simulink model "OutputToVisualizationContinuous"  (R2016b)
settings: Solver=FixedStepDiscrete  StartTime=0.0  StopTime=10.0  FixedStep=sCoreParams.core.stepPeriod  RelTol=1e-3  EnableMultiTasking=on
undefined symbols (not defined in the file): Low, sCoreParams, sCoreParams_viz_channelInds
libraries: dspswit3 x4, simulink x3, xpcrtudplib x2, slrtlib x2, xpcutilitieslib x1, xpcobsoletelib x1
settings Model: DataTypeOverride=Double  MinMaxOverflowLogging=ForceOff  Creator=rzelmann  LastModifiedBy=rzelmann
settings SolverCC: EnableConcurrentExecution=on  ConcurrentTasks=on  AutoInsertRateTranBlk=on
settings DataIOCC: SaveFormat=StructureWithTime  SaveOutput=off  SignalLogging=off  DSMLogging=off  SaveTime=off
settings OptimizationCC: BlockReduction=off  DefaultParameterBehavior=Inlined  LifeSpan=inf
settings DebuggingCC: AllowSymbolicDim=off  SFUnexpectedBacktrackingDiag=warning  SFNoUnconditionalDefaultTransitionDiag=warning  SFExecutionAtInitializationDiag=none
settings HardwareCC: ProdBitPerPointer=32  ProdBitPerSizeT=32  ProdBitPerPtrDiffT=32  ProdLargestAtomicFloat=None  ProdWordSize=32  ProdLongLongMode=on  ProdHWDeviceType=Generic->32-bit x86 compatible
settings ModelReferenceCC: UpdateModelReferenceTargets=Force  ParallelModelReferenceMATLABWorkerInit=Load Top Model  ModelReferenceNumInstancesAllowed=Single  ModelReferencePassRootInputsByReference=off
settings RTWCC: SystemTargetFile=slrt.tlc  TemplateMakefile=slrt_default_tmf  Description=Simulink Real-Time  RTWCompilerOptimization=on
settings CodeAppCC: MaxIdLength=63
settings ConfigComp: CovMetricSettings=dw  CovHtmlReporting=on  CovSaveCumulativeToWorkspaceVar=on  CovSaveSingleToWorkspaceVar=on  CovExternalEMLEnable=off

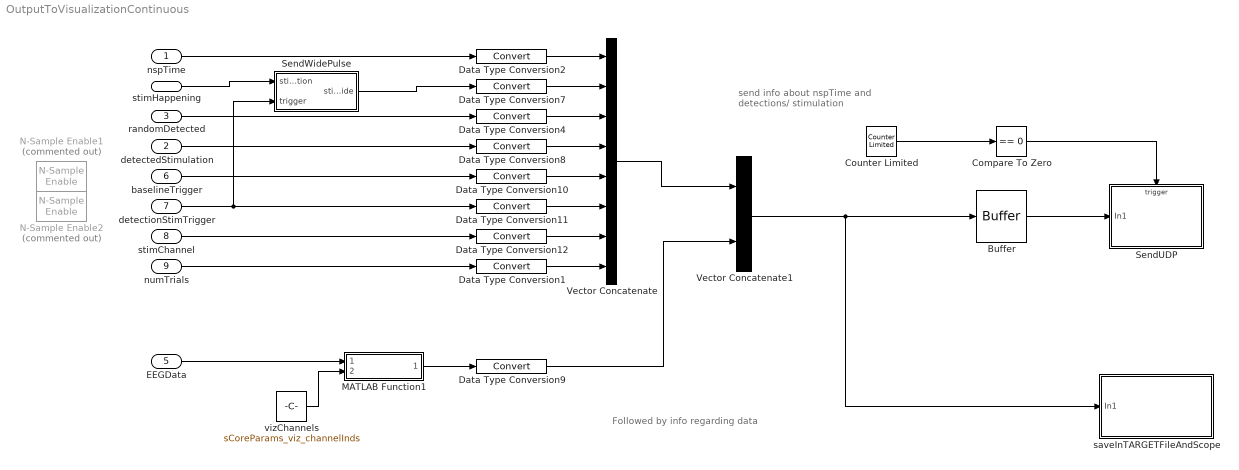
== system OutputToVisualizationContinuous ==
  note: Followed by info regarding data
  note: send info about nspTime
      |  and detections/ stimulation
  nspTime : Inport  SampleTime=sCoreParams.core.stepPeriod
  detectedStimulation : Inport  Port=2  OutDataTypeStr=boolean  SampleTime=sCoreParams.core.stepPeriod
  randomDetected : Inport  Port=3  OutDataTypeStr=boolean  SampleTime=sCoreParams.core.stepPeriod
  stimHappening : Inport  Port=4  OutDataTypeStr=boolean  SampleTime=sCoreParams.core.stepPeriod
  EEGData : Inport  Port=5  PortDimensions=[sCoreParams.core.samplesPerStep sCoreParams.decoders.txDetector.nChannels]  SampleTime=sCoreParams.core.stepPeriod
  baselineTrigger : Inport  Port=6  OutDataTypeStr=int32  SampleTime=sCoreParams.core.stepPeriod  Interpolate=off
  detectionStimTrigger : Inport  Port=7  OutDataTypeStr=int32  SampleTime=sCoreParams.core.stepPeriod  Interpolate=off
  stimChannel : Inport  Port=8  OutDataTypeStr=int32  PortDimensions=[1 2]  SampleTime=sCoreParams.core.stepPeriod  Interpolate=off
  numTrials : Inport  Port=9  SampleTime=sCoreParams.core.stepPeriod
  Buffer : Buffer  N=sCoreParams.write.broadcastSamp  V=sCoreParams.write.broadcastSamp-1  TreatMby1Signals=One channel  OutputFrames=off
  Compare To Zero : simulink/Logic and Bit Operations/Compare To Zero  relop===  OutDataTypeStr=boolean
  Counter Limited : simulink/Sources/Counter Limited  uplimit=sCoreParams.write.broadcastSamp -1  tsamp=sCoreParams.core.stepPeriod
  Data Type Conversion{1..2,4,7..12} (9 alike) : DataTypeConversion
  MATLAB Function1 : MATLAB Function  TreatAsAtomicUnit=on
  N-Sample Enable1 : dspswit3/N-Sample Enable  Commented=on  N=sCoreParams.viz.pulseWidthTriggerSteps  ActiveLevel=Low (0)  reset=on  TriggerType=Rising edge  Ts=1  DataType=Logical
  N-Sample Enable2 : dspswit3/N-Sample Enable  Commented=on  N=sCoreParams.viz.pulseWidthTriggerSteps  ActiveLevel=Low (0)  reset=on  TriggerType=Rising edge  Ts=1  DataType=Logical
  SendUDP : Subsystem
  SendWidePulse : Subsystem
  Vector Concatenate : Concatenate  NumInputs=8
  Vector Concatenate1 : Concatenate
  saveInTARGETFileAndScope : Subsystem
  vizChannels : Constant  Value=sCoreParams_viz_channelInds
  wires:
  Data Type Conversion2/1 -> Vector Concatenate/1
  Counter Limited/1 -> Compare To Zero/1
  Compare To Zero/1 -> SendUDP/Trigger
  Vector Concatenate/1 -> Vector Concatenate1/1
  Data Type Conversion7/1 -> Vector Concatenate/2
  vizChannels/1 -> MATLAB Function1/2(selectCh)
  EEGData/1 -> MATLAB Function1/1(signalIn)
  MATLAB Function1/1(signalOut) -> Data Type Conversion9/1
  Buffer/1 -> SendUDP/1(In1)
  Vector Concatenate1/1 -> saveInTARGETFileAndScope/1(In1), Buffer/1
  stimChannel/1 -> Data Type Conversion12/1
  nspTime/1 -> Data Type Conversion2/1
  numTrials/1 -> Data Type Conversion1/1
  Data Type Conversion4/1 -> Vector Concatenate/3
  Data Type Conversion8/1 -> Vector Concatenate/4
  Data Type Conversion10/1 -> Vector Concatenate/5
  Data Type Conversion11/1 -> Vector Concatenate/6
  Data Type Conversion12/1 -> Vector Concatenate/7
  Data Type Conversion1/1 -> Vector Concatenate/8
  Data Type Conversion9/1 -> Vector Concatenate1/2
  randomDetected/1 -> Data Type Conversion4/1
  detectedStimulation/1 -> Data Type Conversion8/1
  SendWidePulse/1(stimulationWide) -> Data Type Conversion7/1
  baselineTrigger/1 -> Data Type Conversion10/1
  detectionStimTrigger/1 -> Data Type Conversion11/1, SendWidePulse/2(trigger)
  stimHappening/1 -> SendWidePulse/1(stimulation)

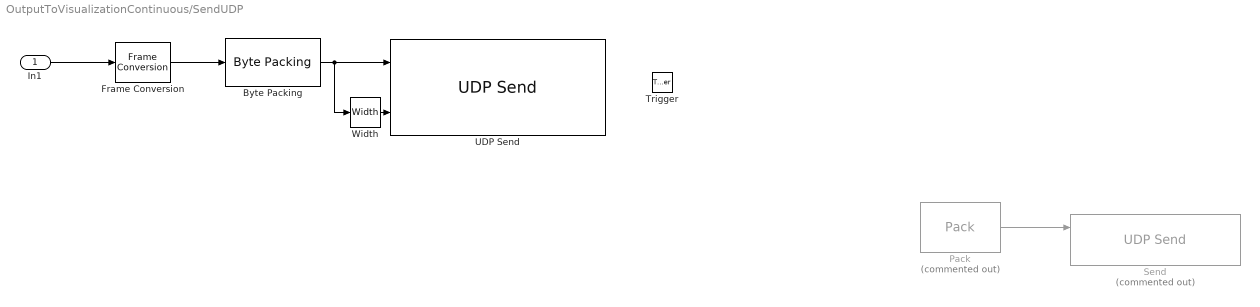
== system OutputToVisualizationContinuous/SendUDP ==
  In1 : Inport
  Trigger : TriggerPort  VariantControl=Variant  PortDimensions=1
  "Byte Packing " : xpcutilitieslib/Byte Packing   MaskPackedDataType=uint8  MaskUnpackedDataTypes={'double'}  MaskAlignment=1
  Frame Conversion : FrameConversion  InheritSamplingMode=off  OutFrame=Sample-based
  Pack : xpcobsoletelib/Utilities/Pack   Commented=on  datatypes={'double'}  byteAlign=1
  Send : xpcrtudplib/UDP Send  Commented=on  ipAddressVal=Use host-target connection  localPort=59121  toAddress=255.255.255.255  toPort=59123  sampleTime=-1
  UDP Send : xpcrtudplib/UDP Send  ipAddressVal=Use host-target connection  localPort=59121  toAddress=255.255.255.255  toPort=59123  sampleTime=-1
  Width : Width
  wires:
  "Byte Packing "/1 -> Width/1, UDP Send/1
  In1/1 -> Frame Conversion/1
  Frame Conversion/1 -> "Byte Packing "/1
  Pack/1 -> Send/1
  Width/1 -> UDP Send/2

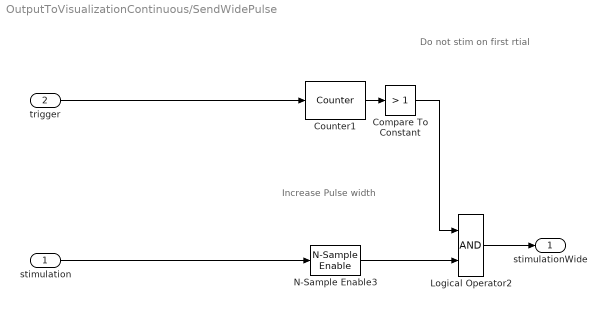
== system OutputToVisualizationContinuous/SendWidePulse ==
  note: Increase Pulse width
  note: Do not stim on first rtial
  stimulation : Inport
  trigger : Inport  Port=2
  Compare To Constant : simulink/Logic and Bit Operations/Compare To Constant  relop=>  const=1  OutDataTypeStr=boolean
  Counter1 : dspswit3/Counter  Direction=Up  CountEvent=Rising edge  CounterSize=16 bits  MaxCount=sCoreParams.decoders.txDetector.detectionDurationSamples  InitialCount=0  Output=Count  HitValue=sCoreParams.decoders.txDetector.detectionDurationSamples  ResetInput=off  SamplesPerFrame=1  Ts=sCoreParams.core.stepPeriod  CntDtype=int32  HitDtype=Logical
  Logical Operator2 : Logic  IconShape=distinctive  AllPortsSameDT=off  OutDataTypeStr=boolean
  N-Sample Enable3 : dspswit3/N-Sample Enable  N=sCoreParams.viz.pulseWidthStimSteps  ActiveLevel=Low (0)  reset=on  TriggerType=Rising edge  Ts=1  DataType=Logical
  stimulationWide : Outport
  wires:
  N-Sample Enable3/1 -> Logical Operator2/2
  Logical Operator2/1 -> stimulationWide/1
  stimulation/1 -> N-Sample Enable3/1
  Counter1/1 -> Compare To Constant/1
  Compare To Constant/1 -> Logical Operator2/1
  trigger/1 -> Counter1/1

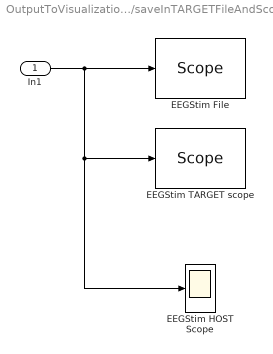
== system OutputToVisualizationContinuous/saveInTARGETFileAndScope ==
  In1 : Inport
  EEGStim File : slrtlib/Displays and Logging/Scope   scopeno=4  scopetype=File  autostart=on  viewmode=Graphical redraw  formatstr='%15.6f'  grid=on  ylimits=[0,0]  nosamples=1000  noprepostsamples=-10  interleave=1  triggermode=FreeRun  triggersignal=1  trigsignalfromport=on  triggerlevel=0.0  triggerslope=Rising  triggerscope=1  triggersample=0  filename=eeg_<%%%>.dat  mode=Lazy  writesize=512  autorestart=on  dynamicfilemode=on  maxwritefilesize=512*1024^2
  EEGStim HOST Scope : Scope
  "EEGStim TARGET scope " : slrtlib/Displays and Logging/Scope   scopeno=5  scopetype=Target  autostart=on  viewmode=Graphical sliding  formatstr='%15.6f'  grid=on  ylimits=[0,0]  nosamples=1000  noprepostsamples=0  interleave=1  triggermode=FreeRun  triggersignal=1  trigsignalfromport=on  triggerlevel=0.0  triggerslope=Rising  triggerscope=1  triggersample=0  filename=data.dat  mode=Lazy  writesize=512  autorestart=off  dynamicfilemode=off  maxwritefilesize=512*1024^2
  wires:
  In1/1 -> EEGStim HOST Scope/1, "EEGStim TARGET scope "/1, EEGStim File/1

== matlab function OutputToVisualizationContinuous/MATLAB Function1 ==
  data: signalIn input; signalOut output size=[1 length(sCoreParams_viz_channelInds)]; selectCh input
function signalOut = selectChannelsFromFrame(signalIn,selectCh)
%#codegen
signalOut = signalIn(end,selectCh); %Only send first time point of frame
%signalOut = selectChannelsFromFrame_EML(signalIn,selectCh);
